simulink model "untitled2121"  (R2016b)
settings: Solver=VariableStepAuto  StartTime=0.0  StopTime=100  FixedStep=1  RelTol=1e-3  SampleTimeConstraint=STIndependent
settings Model: PauseTimes=50  Creator=Administrator  LastModifiedBy=yehoo
settings SolverCC: ShapePreserveControl=EnableAll
settings DataIOCC: LimitDataPoints=on  SaveOutput=off  SaveTime=off
settings OptimizationCC: BlockReduction=off  BooleanDataType=off  LifeSpan=inf
settings DebuggingCC: SaveWithParameterizedLinksMsg=none  UnderspecifiedInitializationDetection=Classic  MergeDetectMultiDrivingBlocksExec=none  SignalResolutionControl=TryResolveAllWithWarning  AllowSymbolicDim=off  SFUnexpectedBacktrackingDiag=warning  SFNoUnconditionalDefaultTransitionDiag=warning  SFExecutionAtInitializationDiag=none
settings HardwareCC: TargetUnknown=on
settings GRTTargetCC: TargetLangStandard=C89/C90 (ANSI)  GeneratePreprocessorConditionals=Disable all
settings ConfigComp: CovMetricSettings=dw  CovHtmlReporting=on  CovSaveCumulativeToWorkspaceVar=on  CovSaveSingleToWorkspaceVar=on  CovExternalEMLEnable=off

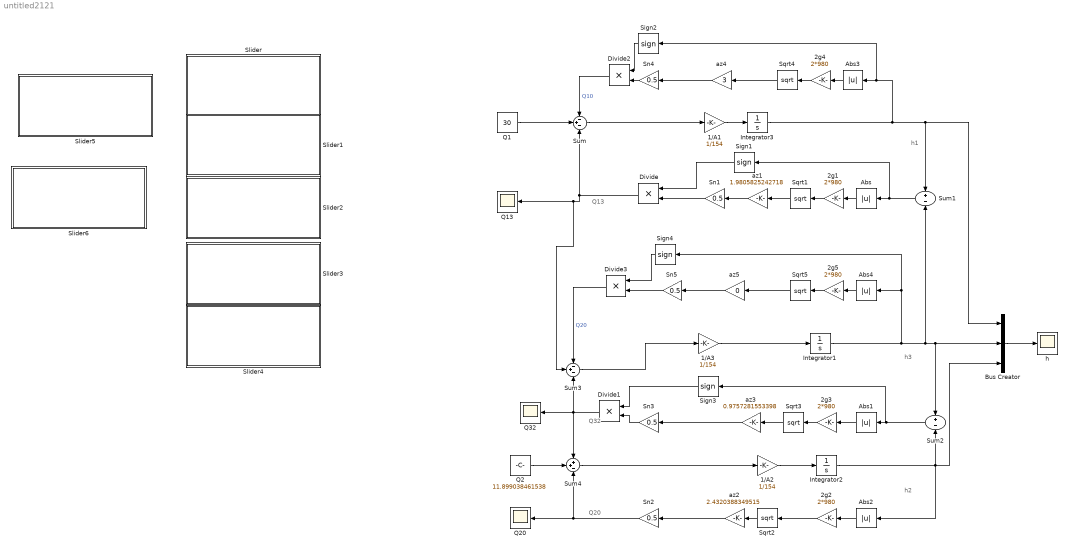
== system untitled2121 ==
  note: Q20
  note: Q32
  note: Q13
  note: h2
  note: h3
  note: h1
  1/A1 : Gain  Gain=1/154
  1/A2 : Gain  Gain=1/154
  1/A3 : Gain  Gain=1/154
  2g{1..5} (5 alike) : Gain  Gain=2*980
  Abs{,1..4} (5 alike) : Abs
  Bus Creator : BusCreator  Inputs=3
  Divide{,1..3} (4 alike) : Product  Inputs=**
  Integrator1 : Integrator
  Integrator2 : Integrator
  Integrator3 : Integrator
  Q1 : Constant  Value=30
  Q13 : Scope
  Q2 : Constant  Value=11.899038461538
  Q20 : Scope
  Q32 : Scope
  Sign{1..4} (4 alike) : Signum
  Slider : Subsystem  DialogController=hmiCreateDDGDialog  IsWebBlock=on  mask(MWDashboardBlock){webBlockId=c4e63f4d-acb7-4280-a73d-de210b8fed9d, webBlockType=slider, ShowInLibBrowser=on, ShowInitialText=on, HMISrcModelName=untitled2121}
      mask prompts: webBlockId "WebBlock Id"; webBlockType "WebBlock Type"; HMISrcModelName "Source Model"
      mask help: SimulinkHMI:dialogs:SliderDialogDesc
      mask Help: helpview([docroot '/mapfiles/simulink.map'], 'hmi_slider')
      mask Display:
      | if strcmp(get_param(bdroot(gcb),'BlockDiagramType'), 'library')
      |     image([(matlabroot) '/toolbox/simulink/hmi/icons/Slider.png']);
      | end
  Slider1 : Subsystem  DialogController=hmiCreateDDGDialog  IsWebBlock=on  mask(MWDashboardBlock){webBlockId=65583228-68c0-41a9-9df9-ab1d7dba6f04, webBlockType=slider, ShowInLibBrowser=on, ShowInitialText=on, HMISrcModelName=untitled2121}
      mask prompts: webBlockId "WebBlock Id"; webBlockType "WebBlock Type"; HMISrcModelName "Source Model"
      mask help: SimulinkHMI:dialogs:SliderDialogDesc
      mask Help: helpview([docroot '/mapfiles/simulink.map'], 'hmi_slider')
      mask Display:
      | if strcmp(get_param(bdroot(gcb),'BlockDiagramType'), 'library')
      |     image([(matlabroot) '/toolbox/simulink/hmi/icons/Slider.png']);
      | end
  Slider2 : Subsystem  DialogController=hmiCreateDDGDialog  IsWebBlock=on  mask(MWDashboardBlock){webBlockId=41a5e724-6674-4671-89ac-82ae44e62c49, webBlockType=slider, ShowInLibBrowser=on, ShowInitialText=on, HMISrcModelName=untitled2121}
      mask prompts: webBlockId "WebBlock Id"; webBlockType "WebBlock Type"; HMISrcModelName "Source Model"
      mask help: SimulinkHMI:dialogs:SliderDialogDesc
      mask Help: helpview([docroot '/mapfiles/simulink.map'], 'hmi_slider')
      mask Display:
      | if strcmp(get_param(bdroot(gcb),'BlockDiagramType'), 'library')
      |     image([(matlabroot) '/toolbox/simulink/hmi/icons/Slider.png']);
      | end
  Slider3 : Subsystem  DialogController=hmiCreateDDGDialog  IsWebBlock=on  mask(MWDashboardBlock){webBlockId=ce634c41-8ecd-43d5-a3b0-a3f2f42860ed, webBlockType=slider, ShowInLibBrowser=on, ShowInitialText=on, HMISrcModelName=untitled2121}
      mask prompts: webBlockId "WebBlock Id"; webBlockType "WebBlock Type"; HMISrcModelName "Source Model"
      mask help: SimulinkHMI:dialogs:SliderDialogDesc
      mask Help: helpview([docroot '/mapfiles/simulink.map'], 'hmi_slider')
      mask Display:
      | if strcmp(get_param(bdroot(gcb),'BlockDiagramType'), 'library')
      |     image([(matlabroot) '/toolbox/simulink/hmi/icons/Slider.png']);
      | end
  Slider4 : Subsystem  DialogController=hmiCreateDDGDialog  IsWebBlock=on  mask(MWDashboardBlock){webBlockId=9cdcea4d-fc7d-41f1-9b2a-1e6e45c895da, webBlockType=slider, ShowInLibBrowser=on, ShowInitialText=on, HMISrcModelName=untitled2121}
      mask prompts: webBlockId "WebBlock Id"; webBlockType "WebBlock Type"; HMISrcModelName "Source Model"
      mask help: SimulinkHMI:dialogs:SliderDialogDesc
      mask Help: helpview([docroot '/mapfiles/simulink.map'], 'hmi_slider')
      mask Display:
      | if strcmp(get_param(bdroot(gcb),'BlockDiagramType'), 'library')
      |     image([(matlabroot) '/toolbox/simulink/hmi/icons/Slider.png']);
      | end
  Slider5 : Subsystem  DialogController=hmiCreateDDGDialog  IsWebBlock=on  mask(MWDashboardBlock){webBlockId=68aa3959-a07d-4211-af96-8cd388c7eac1, webBlockType=slider, ShowInLibBrowser=on, ShowInitialText=on, HMISrcModelName=untitled2121}
      mask prompts: webBlockId "WebBlock Id"; webBlockType "WebBlock Type"; HMISrcModelName "Source Model"
      mask help: SimulinkHMI:dialogs:SliderDialogDesc
      mask Help: helpview([docroot '/mapfiles/simulink.map'], 'hmi_slider')
      mask Display:
      | if strcmp(get_param(bdroot(gcb),'BlockDiagramType'), 'library')
      |     image([(matlabroot) '/toolbox/simulink/hmi/icons/Slider.png']);
      | end
  Slider6 : Subsystem  DialogController=hmiCreateDDGDialog  IsWebBlock=on  mask(MWDashboardBlock){webBlockId=bbdb913d-185a-4671-8c86-d27667b2755b, webBlockType=slider, ShowInLibBrowser=on, ShowInitialText=on, HMISrcModelName=untitled2121}
      mask prompts: webBlockId "WebBlock Id"; webBlockType "WebBlock Type"; HMISrcModelName "Source Model"
      mask help: SimulinkHMI:dialogs:SliderDialogDesc
      mask Help: helpview([docroot '/mapfiles/simulink.map'], 'hmi_slider')
      mask Display:
      | if strcmp(get_param(bdroot(gcb),'BlockDiagramType'), 'library')
      |     image([(matlabroot) '/toolbox/simulink/hmi/icons/Slider.png']);
      | end
  Sn{1..5} (5 alike) : Gain  Gain=0.5
  Sqrt{1..5} (5 alike) : Sqrt  SaturateOnIntegerOverflow=on
  Sum : Sum  Inputs=-+-
  Sum1 : Sum  Inputs=+-
  Sum2 : Sum  Inputs=+-
  Sum3 : Sum  Inputs=-+-
  Sum4 : Sum  Inputs=++-
  az1 : Gain  Gain=1.9805825242718
  az2 : Gain  Gain=2.4320388349515
  az3 : Gain  Gain=0.9757281553398
  az4 : Gain  Gain=3
  az5 : Gain  Gain=0
  h : Scope
  wires:
  Q1/1 -> Sum/2
  az1/1 -> Sn1/1
  Abs/1 -> 2g1/1
  2g1/1 -> Sqrt1/1
  Sqrt1/1 -> az1/1
  Sign1/1 -> Divide/1
  Sn1/1 -> Divide/2
  Divide/1 -> Sum3/2, Q13/1, Sum/3
  az3/1 -> Sn3/1
  Abs1/1 -> 2g3/1
  Sqrt3/1 -> az3/1
  2g3/1 -> Sqrt3/1
  Sign3/1 -> Divide1/1
  Sn3/1 -> Divide1/2
  Divide1/1 -> Sum3/3, Q32/1, Sum4/1
  Sum3/1 -> 1/A3/1
  1/A3/1 -> Integrator1/1
  az2/1 -> Sn2/1
  2g2/1 -> Sqrt2/1
  Sqrt2/1 -> az2/1
  Q2/1 -> Sum4/2
  Sn2/1 -> Sum4/3, Q20/1
  Sum4/1 -> 1/A2/1
  1/A2/1 -> Integrator2/1
  Integrator1/1 -> Sign4/1, Abs4/1, Sum2/1, Bus Creator/2, Sum1/2
  Integrator2/1 -> Bus Creator/3, Sum2/2, Abs2/1
  Sum/1 -> 1/A1/1
  1/A1/1 -> Integrator3/1
  Integrator3/1 -> Sign2/1, Abs3/1, Sum1/1, Bus Creator/1
  Bus Creator/1 -> h/1
  Abs2/1 -> 2g2/1
  az4/1 -> Sn4/1
  Sum1/1 -> Sign1/1, Abs/1
  Abs3/1 -> 2g4/1
  2g4/1 -> Sqrt4/1
  Sqrt4/1 -> az4/1
  Sign2/1 -> Divide2/1
  Sn4/1 -> Divide2/2
  Divide2/1 -> Sum/1  "Q10"
  az5/1 -> Sn5/1
  Sum2/1 -> Sign3/1, Abs1/1
  Abs4/1 -> 2g5/1
  2g5/1 -> Sqrt5/1
  Sqrt5/1 -> az5/1
  Sign4/1 -> Divide3/1
  Sn5/1 -> Divide3/2
  Divide3/1 -> Sum3/1  "Q20"

== system untitled2121/Slider ==

== system untitled2121/Slider1 ==

== system untitled2121/Slider2 ==

== system untitled2121/Slider3 ==

== system untitled2121/Slider4 ==

== system untitled2121/Slider5 ==

== system untitled2121/Slider6 ==
